simulink model "pr2_US_hap"  (R2023b)
settings: Solver=FixedStepAuto  StartTime=0.0  StopTime=inf  FixedStep=Ts  RelTol=1e-3  EnableMultiTasking=on
values from neighbouring files (symbols this model uses):
  b = 100    [params.m]
  den_Gd = Gd.Den{:}    [params.m]
  encoder_scale = 1/12/4 *2*pi    (= 0.1308996939)    [params.m]
  f = 100    [params.m]
  J = 0.02    [params.m]
  Kb = 0.1    [params.m]
  KD = 0    [params.m]
  Kf = 0.01    [params.m]
  KI = 0.2    [params.m]
  Km = 1    [params.m]
  KP = 0.05    [params.m]
  l = 100    [params.m]
  L = 0.5    [params.m]
  num_Gd = Gd.Num{:}    [params.m]
  r = 100    [params.m]
  R = 2.0    (= 2)    [params.m]
  Vlim = 12    [params.m]
libraries: arduinolib x9, arduinosensorlib x7, simulink x3
settings Model: ExtModeTrigDuration=2  Creator=ghkdt  LastModifiedBy=SJ
settings SolverCC: AutoInsertRateTranBlk=on
settings OptimizationCC: EnhancedBackFolding=on  PassReuseOutputArgsAs=Individual arguments  ZeroExternalMemoryAtStartup=off  ZeroInternalMemoryAtStartup=off  MaxStackSize=64  OptimizeBlockOrder=speed  DifferentSizesBufferReuse=on  OptimizationCustomize=off  EfficientTunableParamExpr=on
settings DebuggingCC: ParameterTunabilityLossMsg=error
settings HardwareCC: ProdBitPerInt=16  ProdBitPerPointer=16  ProdBitPerSizeT=16  ProdBitPerPtrDiffT=16  ProdLargestAtomicFloat=None  ProdWordSize=8  ProdHWDeviceType=Atmel->AVR
settings SFSimCC: MATLABDynamicMemAlloc=off
settings RTWCC: Description=Embedded Coder  SystemTargetFile=ert.tlc  HardwareBoard=Arduino Mega 2560  TemplateMakefile=ert_default_tmf  Toolchain=Arduino AVR  BuildConfiguration=Faster Runs
settings CodeAppCC: ForceParamTrailComments=on  IgnoreCustomStorageClasses=off  OperatorAnnotations=on  SimulinkDataObjDesc=on  SFDataObjDesc=on  InsertBlockDesc=on
settings ERTTargetCC: SupportContinuousTime=on  SupportVariableSizeSignals=on  ExtModeTransport=3  ExtModeStaticAlloc=on  ExtModeAutomaticAllocSize=off  ExtModeStaticAllocSize=2048  ExtModeMexFile=ext_xcp  ExtModeIntrfLevel=Level2 - Open

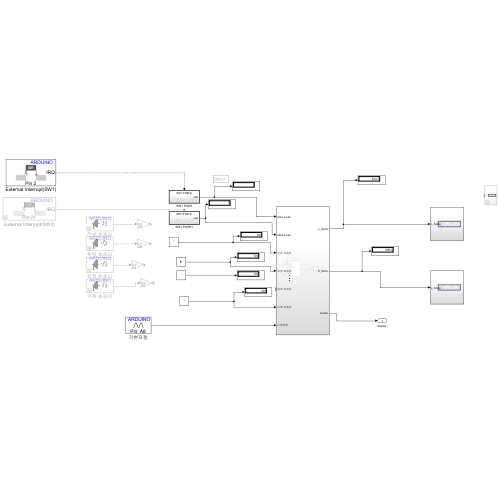
[thumbnail: Simulink's stored preview of the top-level diagram]
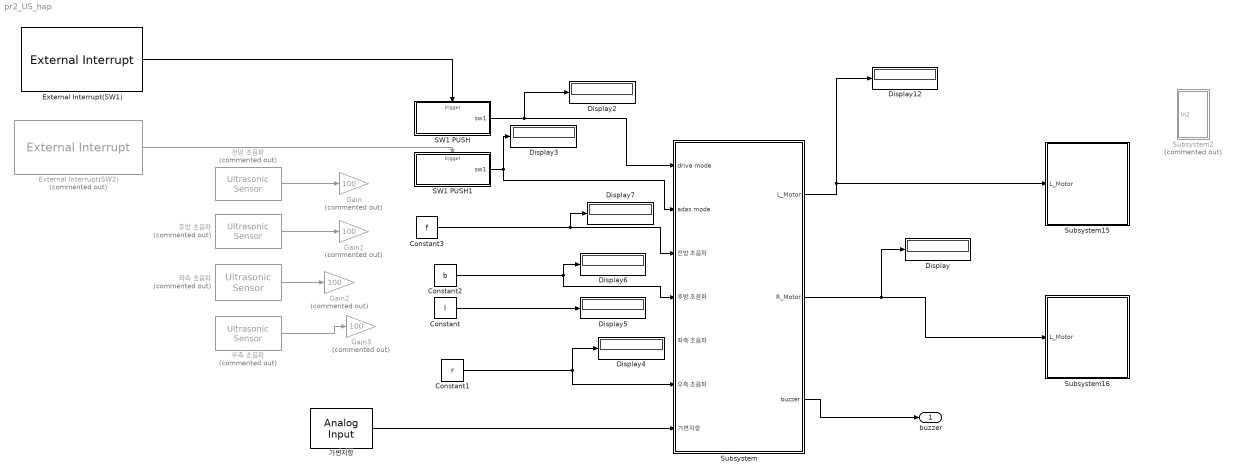
== system pr2_US_hap ==
  Constant : Constant  Value=l
  Constant1 : Constant  Value=r
  Constant2 : Constant  Value=b
  Constant3 : Constant  Value=f
  Display{,2..7,12} (8 alike) : Display
  External Interrupt(SW1) : arduinolib/External Interrupt  Pin=2  PullUp=off  Mode=RISING  InterruptSimulationInput=off
  External Interrupt(SW2) : arduinolib/External Interrupt  Commented=on  Pin=21  PullUp=off  Mode=RISING  InterruptSimulationInput=off
  Gain{,1..3} (4 alike) : Gain  Commented=on  Gain=100
  SW1 PUSH : Subsystem  TreatAsAtomicUnit=on
  SW1 PUSH1 : Subsystem  TreatAsAtomicUnit=on
  Subsystem : Subsystem
  Subsystem15 : Subsystem
  Subsystem16 : Subsystem
  Subsystem2 : Subsystem  Commented=on
  가변저항 : arduinolib/Analog Input  pinNumber=8  ReadResultsOnly=off  ConversionTriggerSource=Software  ExternalTriggerType=uint32( 0 )  OutputDataType=uint16  EnableConversionCompleteNotify=off  EnableOuputStatus=off  SampleTime=-1  blockPlatform=arduino
  우측 초음파 : arduinosensorlib/Ultrasonic Sensor  Commented=on  NumSignalPins=2  TrigPin=52  EchoPin=53  SignalPin=3  SampleTime_=0.1  blockPlatform=ARDUINO
  전방 초음파 : arduinosensorlib/Ultrasonic Sensor  Commented=on  NumSignalPins=2  TrigPin=46  EchoPin=47  SignalPin=3  SampleTime_=0.1  blockPlatform=ARDUINO
  좌측 초음파 : arduinosensorlib/Ultrasonic Sensor  Commented=on  NumSignalPins=2  TrigPin=50  EchoPin=51  SignalPin=3  SampleTime_=0.1  blockPlatform=ARDUINO
  후방 초음파 : arduinosensorlib/Ultrasonic Sensor  Commented=on  NumSignalPins=2  TrigPin=48  EchoPin=49  SignalPin=3  SampleTime_=0.1  blockPlatform=ARDUINO
  buzzer : Outport
  wires:
  Subsystem/1(L_Motor) -> Subsystem15/1(L_Motor), Display12/1
  SW1 PUSH1/1(sw1) -> Subsystem/2(adas mode), Display3/1
  SW1 PUSH/1(sw1) -> Subsystem/1(drive mode), Display2/1
  가변저항/1 -> Subsystem/7(가변저항)
  Subsystem/3(buzzer) -> buzzer/1
  External Interrupt(SW1)/1 -> SW1 PUSH/Trigger
  External Interrupt(SW2)/1 -> SW1 PUSH1/Trigger
  Constant2/1 -> Subsystem/4(후방 초음파), Display6/1
  Constant1/1 -> Subsystem/6(우측 초음파), Display4/1
  Constant3/1 -> Subsystem/3(전방 초음파), Display7/1
  후방 초음파/1 -> Gain1/1
  우측 초음파/1 -> Gain3/1
  좌측 초음파/1 -> Gain2/1
  전방 초음파/1 -> Gain/1
  Constant/1 -> Display5/1
  Subsystem/2(R_Motor) -> Display/1, Subsystem16/1(L_Motor)

== system pr2_US_hap/SW1 PUSH ==
  SW1 PUSH : TriggerPort  TriggerType=function-call  VariantControl=(inherit)
  Add : Sum  Inputs=+-
  Constant : Constant
  Delay : Delay  DelayLength=1
  sw1 : Outport
  wires:
  Delay/1 -> Add/2
  Add/1 -> sw1/1, Delay/1
  Constant/1 -> Add/1

== system pr2_US_hap/SW1 PUSH1 ==
  SW1 PUSH : TriggerPort  TriggerType=function-call  VariantControl=(inherit)
  Add : Sum  Inputs=+-
  Constant : Constant
  Delay : Delay  DelayLength=1
  sw1 : Outport
  wires:
  Delay/1 -> Add/2
  Add/1 -> sw1/1, Delay/1
  Constant/1 -> Add/1

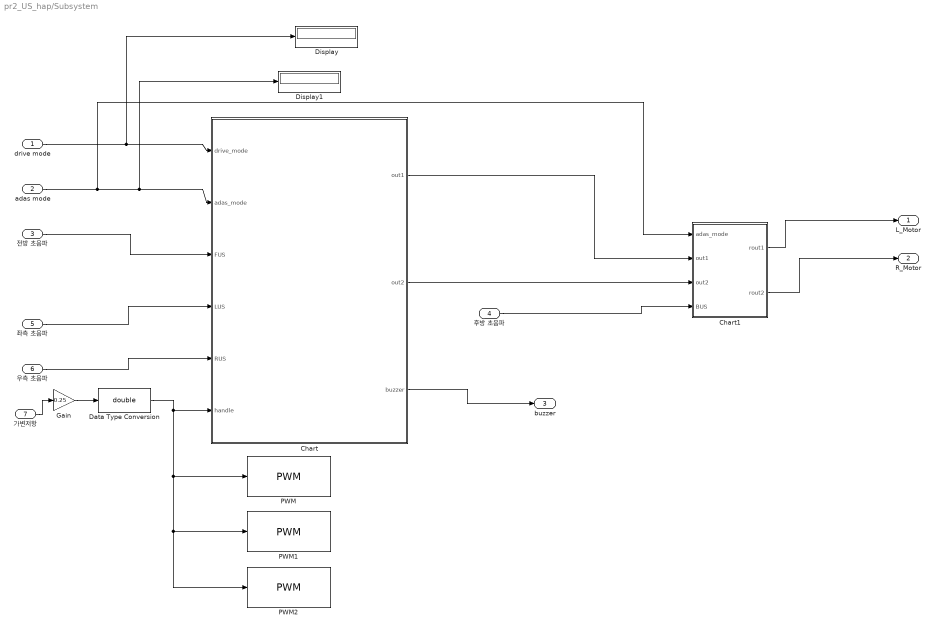
== system pr2_US_hap/Subsystem ==
  drive mode : Inport
  adas mode : Inport  Port=2
  전방 초음파 : Inport  Port=3
  후방 초음파 : Inport  Port=4
  좌측 초음파 : Inport  Port=5
  우측 초음파 : Inport  Port=6
  가변저항 : Inport  Port=7
  Chart : Stateflow chart  TreatAsAtomicUnit=on
  Chart1 : Stateflow chart  TreatAsAtomicUnit=on
  Data Type Conversion : DataTypeConversion  OutDataTypeStr=double  SaturateOnIntegerOverflow=off  RndMeth=Floor
  Display : Display
  Display1 : Display
  Gain : Gain  Gain=0.25
  PWM : arduinolib/PWM  pinNumber=RGB_LED_1  frequencyType=Default  desiredFrequency=490.2  achievableFrequency=490.2
  PWM1 : arduinolib/PWM  pinNumber=RGB_LED_2  frequencyType=Default  desiredFrequency=490.2  achievableFrequency=490.2
  PWM2 : arduinolib/PWM  pinNumber=RGB_LED_3  frequencyType=Default  desiredFrequency=490.2  achievableFrequency=490.2
  L_Motor : Outport
  R_Motor : Outport  Port=2
  buzzer : Outport  Port=3
  wires:
  drive mode/1 -> Chart/1(drive_mode), Display/1
  adas mode/1 -> Chart1/1(adas_mode), Chart/2(adas_mode), Display1/1
  전방 초음파/1 -> Chart/3(FUS)
  후방 초음파/1 -> Chart1/4(BUS)
  좌측 초음파/1 -> Chart/4(LUS)
  우측 초음파/1 -> Chart/5(RUS)
  Chart/3(buzzer) -> buzzer/1
  Chart/1(out1) -> Chart1/2(out1)
  Chart/2(out2) -> Chart1/3(out2)
  Chart1/1(rout1) -> L_Motor/1
  Chart1/2(rout2) -> R_Motor/1
  가변저항/1 -> Gain/1
  Gain/1 -> Data Type Conversion/1
  Data Type Conversion/1 -> PWM2/1, PWM1/1, PWM/1, Chart/6(handle)

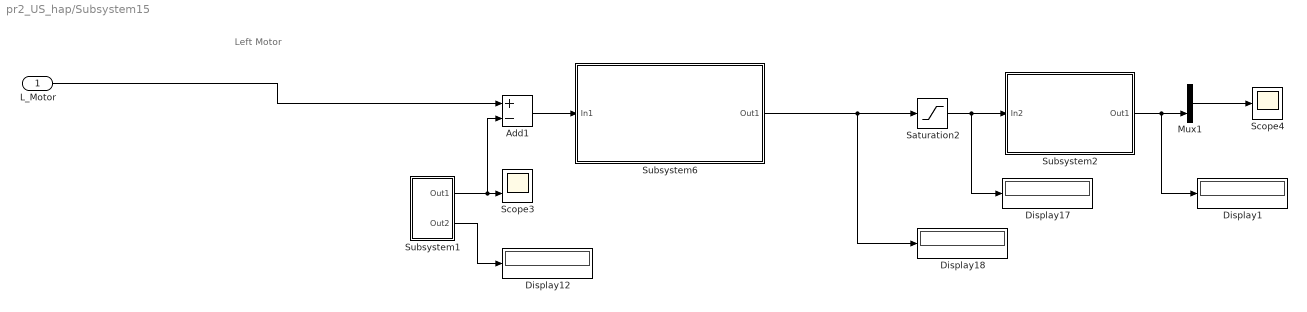
== system pr2_US_hap/Subsystem15 ==
  note: Left Motor
  L_Motor : Inport
  Add1 : Sum  Inputs=+-
  Display{1,12,17..18} (4 alike) : Display
  Mux1 : Mux  Inputs=2
  Saturation2 : Saturate  UpperLimit=12  LowerLimit=0
  Scope3 : Scope  NumInputPorts=2
  Scope4 : Scope
  Subsystem1 : Subsystem
  Subsystem2 : Subsystem
  Subsystem6 : Subsystem
  wires:
  Subsystem2/1(Out1) -> Display1/1, Mux1/2
  Subsystem1/2(Out2) -> Display12/1
  Subsystem6/1(Out1) -> Display18/1, Saturation2/1
  Add1/1 -> Subsystem6/1(In1)
  Mux1/1 -> Scope4/1
  Subsystem1/1(Out1) -> Add1/2, Scope3/2
  Saturation2/1 -> Subsystem2/1(In2), Display17/1
  L_Motor/1 -> Add1/1

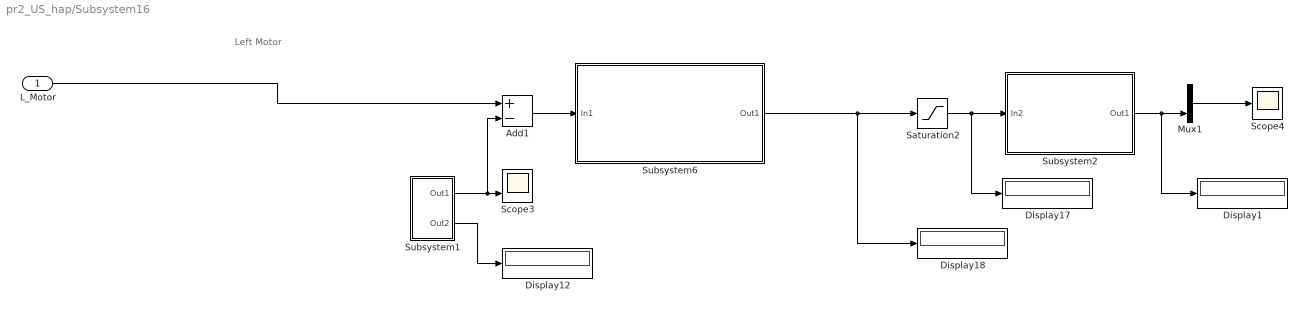
== system pr2_US_hap/Subsystem16 ==
  note: Left Motor
  L_Motor : Inport
  Add1 : Sum  Inputs=+-
  Display{1,12,17..18} (4 alike) : Display
  Mux1 : Mux  Inputs=2
  Saturation2 : Saturate  UpperLimit=12  LowerLimit=0
  Scope3 : Scope  NumInputPorts=2
  Scope4 : Scope
  Subsystem1 : Subsystem
  Subsystem2 : Subsystem
  Subsystem6 : Subsystem
  wires:
  Subsystem2/1(Out1) -> Display1/1, Mux1/2
  Subsystem1/2(Out2) -> Display12/1
  Subsystem6/1(Out1) -> Display18/1, Saturation2/1
  Add1/1 -> Subsystem6/1(In1)
  Mux1/1 -> Scope4/1
  Subsystem1/1(Out1) -> Add1/2, Scope3/2
  Saturation2/1 -> Subsystem2/1(In2), Display17/1
  L_Motor/1 -> Add1/1

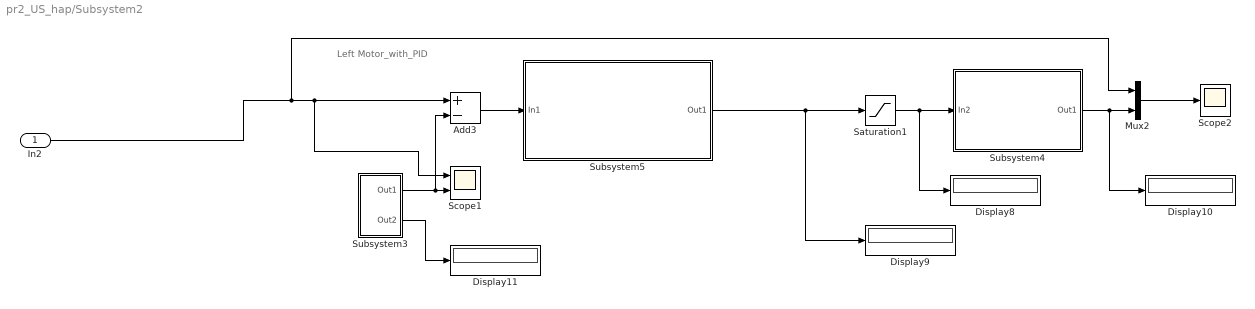
== system pr2_US_hap/Subsystem2 ==
  note: Left Motor_with_PID
  In2 : Inport
  Add3 : Sum  Inputs=+-
  Display{8..11} (4 alike) : Display
  Mux2 : Mux  Inputs=2
  Saturation1 : Saturate  UpperLimit=12  LowerLimit=0
  Scope1 : Scope  NumInputPorts=2
  Scope2 : Scope
  Subsystem3 : Subsystem
  Subsystem4 : Subsystem
  Subsystem5 : Subsystem
  wires:
  Mux2/1 -> Scope2/1
  Saturation1/1 -> Subsystem4/1(In2), Display8/1
  Subsystem5/1(Out1) -> Display9/1, Saturation1/1
  Subsystem3/1(Out1) -> Add3/2, Scope1/2
  Subsystem3/2(Out2) -> Display11/1
  Add3/1 -> Subsystem5/1(In1)
  Subsystem4/1(Out1) -> Display10/1, Mux2/2
  In2/1 -> Mux2/1, Scope1/1, Add3/1

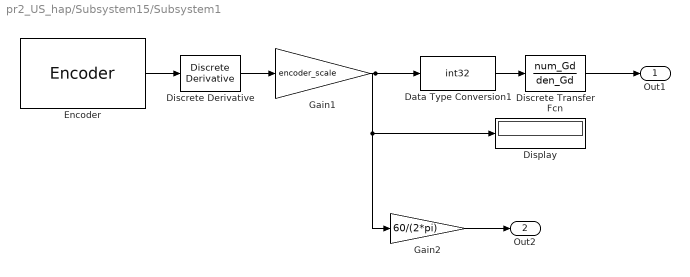
== system pr2_US_hap/Subsystem15/Subsystem1 ==
  Data Type Conversion1 : DataTypeConversion  OutDataTypeStr=int32  SaturateOnIntegerOverflow=off  RndMeth=Floor
  Discrete Transfer Fcn : DiscreteTransferFcn  Numerator=num_Gd  Denominator=den_Gd
  Discrete Derivative : simulink/Discrete/Discrete Derivative  gainval=1.0  ICPrevScaledInput=0.0  OutMin=[]  OutMax=[]  OutDataType=fixdt(1, 16)  OutScaling=2^-10  DoSatur=off
  Display : Display
  Encoder : arduinosensorlib/Encoder  InputA=18  InputB=19  Mode=No reset  SampleTime=-1
  Gain1 : Gain  Gain=encoder_scale
  Gain2 : Gain  Gain=60/(2*pi)
  Out1 : Outport
  Out2 : Outport  Port=2
  wires:
  Gain1/1 -> Display/1, Gain2/1, Data Type Conversion1/1
  Encoder/1 -> Discrete Derivative/1
  Gain2/1 -> Out2/1
  Data Type Conversion1/1 -> Discrete Transfer Fcn/1
  Discrete Derivative/1 -> Gain1/1
  Discrete Transfer Fcn/1 -> Out1/1

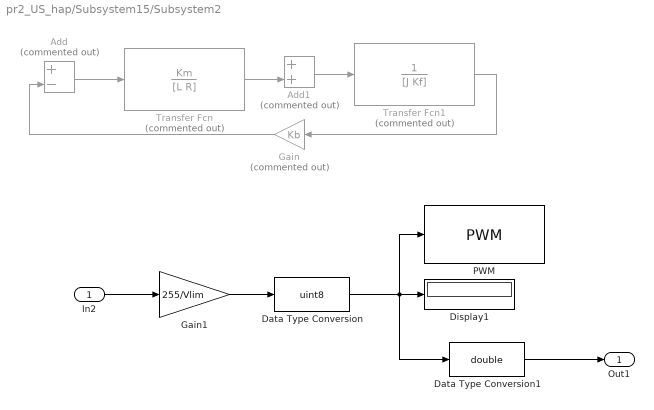
== system pr2_US_hap/Subsystem15/Subsystem2 ==
  In2 : Inport
  Add : Sum  Commented=on  Inputs=+-
  Add1 : Sum  Commented=on
  Data Type Conversion : DataTypeConversion  OutDataTypeStr=uint8  SaturateOnIntegerOverflow=off  RndMeth=Floor
  Data Type Conversion1 : DataTypeConversion  OutDataTypeStr=double  SaturateOnIntegerOverflow=off  RndMeth=Floor
  Display1 : Display
  Gain : Gain  Commented=on  Gain=Kb
  Gain1 : Gain  Gain=255/Vlim
  PWM : arduinolib/PWM  pinNumber=11  frequencyType=Default  desiredFrequency=490.2  achievableFrequency=490.2
  Transfer Fcn : TransferFcn  Commented=on  Numerator=Km  Denominator=[L R]
  Transfer Fcn1 : TransferFcn  Commented=on  Numerator=1  Denominator=[J Kf]
  Out1 : Outport
  wires:
  ? -> Add/1
  ? -> Add1/1
  Add/1 -> Transfer Fcn/1
  Add1/1 -> Transfer Fcn1/1
  Transfer Fcn/1 -> Add1/2
  Gain/1 -> Add/2
  Transfer Fcn1/1 -> Gain/1
  In2/1 -> Gain1/1
  Gain1/1 -> Data Type Conversion/1
  Data Type Conversion1/1 -> Out1/1
  Data Type Conversion/1 -> Data Type Conversion1/1, Display1/1, PWM/1

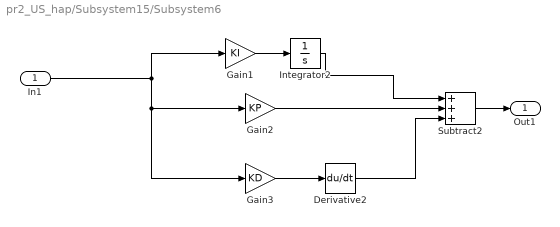
== system pr2_US_hap/Subsystem15/Subsystem6 ==
  In1 : Inport
  Derivative2 : Derivative
  Gain1 : Gain  Gain=KI
  Gain2 : Gain  Gain=KP
  Gain3 : Gain  Gain=KD
  Integrator2 : Integrator
  Subtract2 : Sum  Inputs=+++
  Out1 : Outport
  wires:
  Gain1/1 -> Integrator2/1
  Gain2/1 -> Subtract2/2
  Integrator2/1 -> Subtract2/1
  In1/1 -> Gain2/1, Gain3/1, Gain1/1
  Derivative2/1 -> Subtract2/3
  Gain3/1 -> Derivative2/1
  Subtract2/1 -> Out1/1

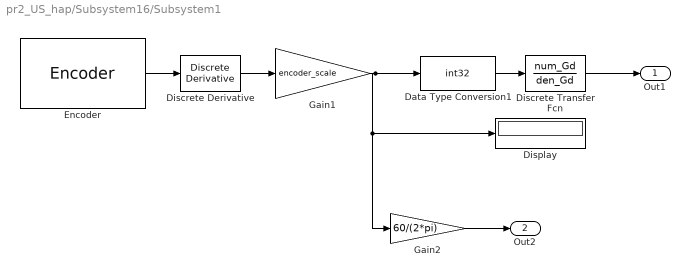
== system pr2_US_hap/Subsystem16/Subsystem1 ==
  Data Type Conversion1 : DataTypeConversion  OutDataTypeStr=int32  SaturateOnIntegerOverflow=off  RndMeth=Floor
  Discrete Transfer Fcn : DiscreteTransferFcn  Numerator=num_Gd  Denominator=den_Gd
  Discrete Derivative : simulink/Discrete/Discrete Derivative  gainval=1.0  ICPrevScaledInput=0.0  OutMin=[]  OutMax=[]  OutDataType=fixdt(1, 16)  OutScaling=2^-10  DoSatur=off
  Display : Display
  Encoder : arduinosensorlib/Encoder  InputA=20  InputB=21  Mode=No reset  SampleTime=-1
  Gain1 : Gain  Gain=encoder_scale
  Gain2 : Gain  Gain=60/(2*pi)
  Out1 : Outport
  Out2 : Outport  Port=2
  wires:
  Gain1/1 -> Display/1, Gain2/1, Data Type Conversion1/1
  Encoder/1 -> Discrete Derivative/1
  Gain2/1 -> Out2/1
  Data Type Conversion1/1 -> Discrete Transfer Fcn/1
  Discrete Derivative/1 -> Gain1/1
  Discrete Transfer Fcn/1 -> Out1/1

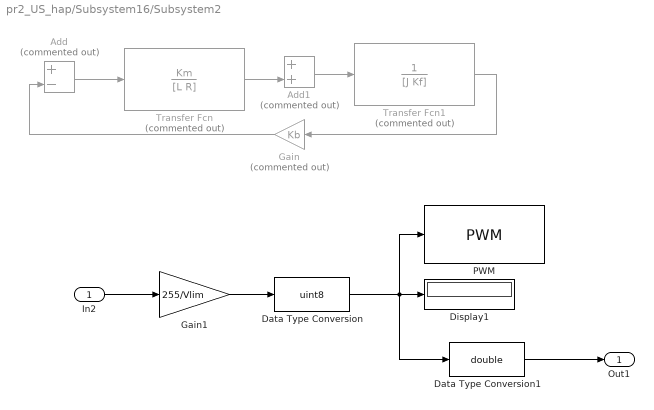
== system pr2_US_hap/Subsystem16/Subsystem2 ==
  In2 : Inport
  Add : Sum  Commented=on  Inputs=+-
  Add1 : Sum  Commented=on
  Data Type Conversion : DataTypeConversion  OutDataTypeStr=uint8  SaturateOnIntegerOverflow=off  RndMeth=Floor
  Data Type Conversion1 : DataTypeConversion  OutDataTypeStr=double  SaturateOnIntegerOverflow=off  RndMeth=Floor
  Display1 : Display
  Gain : Gain  Commented=on  Gain=Kb
  Gain1 : Gain  Gain=255/Vlim
  PWM : arduinolib/PWM  pinNumber=3  frequencyType=Default  desiredFrequency=490.2  achievableFrequency=490.2
  Transfer Fcn : TransferFcn  Commented=on  Numerator=Km  Denominator=[L R]
  Transfer Fcn1 : TransferFcn  Commented=on  Numerator=1  Denominator=[J Kf]
  Out1 : Outport
  wires:
  ? -> Add/1
  ? -> Add1/1
  Add/1 -> Transfer Fcn/1
  Add1/1 -> Transfer Fcn1/1
  Transfer Fcn/1 -> Add1/2
  Gain/1 -> Add/2
  Transfer Fcn1/1 -> Gain/1
  In2/1 -> Gain1/1
  Gain1/1 -> Data Type Conversion/1
  Data Type Conversion1/1 -> Out1/1
  Data Type Conversion/1 -> Data Type Conversion1/1, Display1/1, PWM/1

== system pr2_US_hap/Subsystem16/Subsystem6 ==
  In1 : Inport
  Derivative2 : Derivative
  Gain1 : Gain  Gain=KI
  Gain2 : Gain  Gain=KP
  Gain3 : Gain  Gain=KD
  Integrator2 : Integrator
  Subtract2 : Sum  Inputs=+++
  Out1 : Outport
  wires:
  Gain1/1 -> Integrator2/1
  Gain2/1 -> Subtract2/2
  Integrator2/1 -> Subtract2/1
  In1/1 -> Gain2/1, Gain3/1, Gain1/1
  Derivative2/1 -> Subtract2/3
  Gain3/1 -> Derivative2/1
  Subtract2/1 -> Out1/1

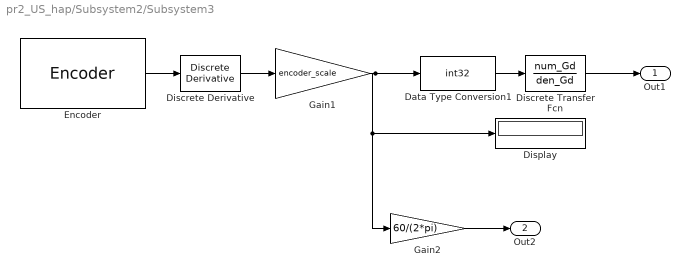
== system pr2_US_hap/Subsystem2/Subsystem3 ==
  Data Type Conversion1 : DataTypeConversion  OutDataTypeStr=int32  SaturateOnIntegerOverflow=off  RndMeth=Floor
  Discrete Transfer Fcn : DiscreteTransferFcn  Numerator=num_Gd  Denominator=den_Gd
  Discrete Derivative : simulink/Discrete/Discrete Derivative  gainval=1.0  ICPrevScaledInput=0.0  OutMin=[]  OutMax=[]  OutDataType=fixdt(1, 16)  OutScaling=2^-10  DoSatur=off
  Display : Display
  Encoder : arduinosensorlib/Encoder  InputA=18  InputB=19  Mode=No reset  SampleTime=-1
  Gain1 : Gain  Gain=encoder_scale
  Gain2 : Gain  Gain=60/(2*pi)
  Out1 : Outport
  Out2 : Outport  Port=2
  wires:
  Gain1/1 -> Display/1, Gain2/1, Data Type Conversion1/1
  Encoder/1 -> Discrete Derivative/1
  Gain2/1 -> Out2/1
  Data Type Conversion1/1 -> Discrete Transfer Fcn/1
  Discrete Derivative/1 -> Gain1/1
  Discrete Transfer Fcn/1 -> Out1/1

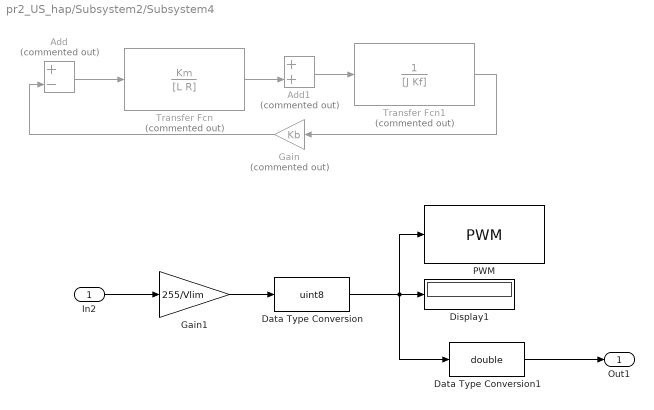
== system pr2_US_hap/Subsystem2/Subsystem4 ==
  In2 : Inport
  Add : Sum  Commented=on  Inputs=+-
  Add1 : Sum  Commented=on
  Data Type Conversion : DataTypeConversion  OutDataTypeStr=uint8  SaturateOnIntegerOverflow=off  RndMeth=Floor
  Data Type Conversion1 : DataTypeConversion  OutDataTypeStr=double  SaturateOnIntegerOverflow=off  RndMeth=Floor
  Display1 : Display
  Gain : Gain  Commented=on  Gain=Kb
  Gain1 : Gain  Gain=255/Vlim
  PWM : arduinolib/PWM  pinNumber=11  frequencyType=Default  desiredFrequency=490.2  achievableFrequency=490.2
  Transfer Fcn : TransferFcn  Commented=on  Numerator=Km  Denominator=[L R]
  Transfer Fcn1 : TransferFcn  Commented=on  Numerator=1  Denominator=[J Kf]
  Out1 : Outport
  wires:
  ? -> Add/1
  ? -> Add1/1
  Add/1 -> Transfer Fcn/1
  Add1/1 -> Transfer Fcn1/1
  Transfer Fcn/1 -> Add1/2
  Gain/1 -> Add/2
  Transfer Fcn1/1 -> Gain/1
  In2/1 -> Gain1/1
  Gain1/1 -> Data Type Conversion/1
  Data Type Conversion1/1 -> Out1/1
  Data Type Conversion/1 -> Data Type Conversion1/1, Display1/1, PWM/1

== system pr2_US_hap/Subsystem2/Subsystem5 ==
  In1 : Inport
  Derivative2 : Derivative
  Gain1 : Gain  Gain=KI
  Gain2 : Gain  Gain=KP
  Gain3 : Gain  Gain=KD
  Integrator2 : Integrator
  Subtract2 : Sum  Inputs=+++
  Out1 : Outport
  wires:
  Gain1/1 -> Integrator2/1
  Gain2/1 -> Subtract2/2
  Integrator2/1 -> Subtract2/1
  In1/1 -> Gain2/1, Gain3/1, Gain1/1
  Derivative2/1 -> Subtract2/3
  Gain3/1 -> Derivative2/1
  Subtract2/1 -> Out1/1

== stateflow chart pr2_US_hap/Subsystem/Chart1 ==
  state adas_off
    en,du:
    rout1=out1;
    rout2=out2;
  state adas_on
    en,du:
    rout1=out1;
    rout2=out2;
  state adas_on_BUS
    en,du:
    rout1=out1*1.2;
    rout2=out2*1.2;
  adas_on_BUS -> adas_off [order 2] : [adas_mode==0]
  (default) -> adas_off
  adas_on -> adas_on_BUS [order 2] : [BUS<=10]
  adas_off -> adas_on : [adas_mode==1]
  adas_on -> adas_off [order 1] : [adas_mode==0]
  adas_on_BUS -> adas_on [order 1] : [BUS>10]
  data: adas_mode input; out1 input; out2 input; BUS input; rout1 output; rout2 output

== stateflow chart pr2_US_hap/Subsystem/Chart ==
  state drive_on_adas_on
    en, du:
    out1 = default;
    out2 = default;
  state drive_off
    en, du:
    out1 = 0;
    out2 = 0;
    steering = 0.02;
    default = 360;
  state drive_on_adas_off
    en, du:
    out1 = default*(1+(handle-128)/6.4/100);
    out2 = default*(1+(128-handle)/6.4/100);
    exit:
    buzzer = 0;
  state drive_on_adas_on_FUS
    en,du:
    out1 = 0;
    out2 = 0;
    buzzer = 1;
    exit:
    buzzer = 0;
  state drive_on_adas_on_LUS
    en,du:
    out1 = default*(1+(10-LUS)*steering);
    out2 = default*(1-(10-LUS)*steering);
  state drive_on_adas_on_RUS
    en,du:
    out1 = default*(1-(10-RUS)*steering);
    out2 = default*(1+(10-RUS)*steering);
  state drive_on_adas_on_LRUS
    en,du:
    out1 = default*(1-(LUS-RUS)*steering);
    out2 = default*(1+(LUS-RUS)*steering);
  drive_on_adas_on_FUS -> drive_on_adas_off [order 5] : [adas_mode ==0]
  (default) -> drive_off
  drive_on_adas_on -> drive_on_adas_on_FUS [order 2] : [FUS<=10]
  drive_on_adas_on_FUS -> drive_on_adas_on_LUS [order 4] : [LUS<=10&&FUS>10]
  drive_off -> drive_on_adas_off : [drive_mode==1]
  drive_on_adas_off -> drive_on_adas_on [order 2] : [adas_mode == 1]
  drive_on_adas_on_FUS -> drive_on_adas_on [order 1] : [LUS>10&&RUS>10&&FUS>10]
  drive_on_adas_off -> drive_off [order 1] : [drive_mode ==0]
  drive_on_adas_on_FUS -> drive_on_adas_on_LRUS [order 2] : [LUS<=10&&RUS<=10&&FUS>10]
  drive_on_adas_on -> drive_on_adas_off [order 1] : [adas_mode  == 0]
  drive_on_adas_on_RUS -> drive_on_adas_off [order 4] : [adas_mode ==0]
  drive_on_adas_on -> drive_on_adas_on_LUS [order 4] : [LUS<=10]
  drive_on_adas_on_LUS -> drive_on_adas_on [order 1] : [LUS>10]
  drive_on_adas_on -> drive_on_adas_on_RUS [order 3] : [RUS<=10]
  drive_on_adas_on_RUS -> drive_on_adas_on [order 1] : [RUS>10]
  drive_on_adas_on_LUS -> drive_on_adas_off [order 4] : [adas_mode ==0]
  drive_on_adas_on_LRUS -> drive_on_adas_off [order 4] : [adas_mode==0]
  drive_on_adas_on_LUS -> drive_on_adas_on_FUS [order 3] : [FUS<=10]
  drive_on_adas_on_LRUS -> drive_on_adas_on_FUS [order 1] : [FUS<=10]
  drive_on_adas_on_RUS -> drive_on_adas_on_FUS [order 2] : [FUS<=10]
  drive_on_adas_on_FUS -> drive_on_adas_on_RUS [order 3] : [RUS<=10&&FUS>10]
  drive_on_adas_on_RUS -> drive_on_adas_on_LRUS [order 3] : [LUS<=10]
  drive_on_adas_on_LRUS -> drive_on_adas_on_RUS [order 3] : [LUS>10]
  drive_on_adas_on_LUS -> drive_on_adas_on_LRUS [order 2] : [RUS<=10]
  drive_on_adas_on_LRUS -> drive_on_adas_on_LUS [order 2] : [RUS>10]
  data: drive_mode input; adas_mode input; FUS input; LUS input; RUS input; out1 output; out2 output; handle input double; buzzer output; steering local double; speed1 local double; speed2 local double; default local double
